simulink model "pompa_cu_perturbatie"  (R2022b)
settings: Solver=VariableStepAuto  StartTime=0.0  StopTime=10.0  RelTol=1e-3
values from neighbouring files (symbols this model uses):
  k = 0.043    [run_first.m]
  k2 = -0.015    [run_first.m]
settings Model: Creator=fabian  LastModifiedBy=fabian

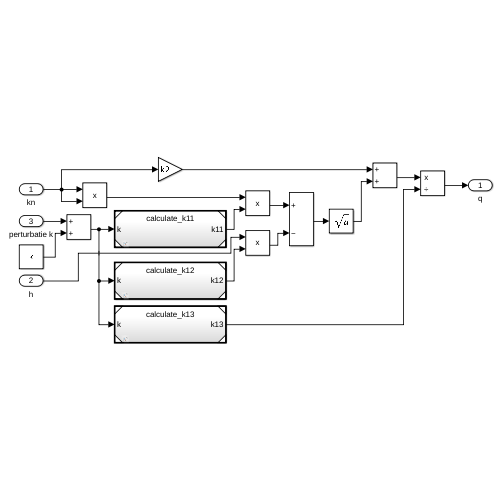
[thumbnail: Simulink's stored preview of the top-level diagram]
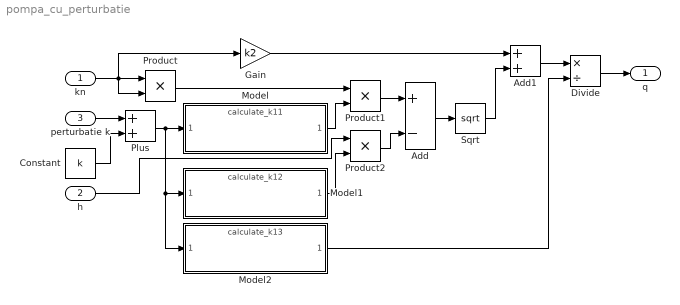
== system pompa_cu_perturbatie ==
  kn : Inport
  h : Inport  Port=2
  perturbatie k : Inport  Port=3
  Add : Sum  Inputs=+-
  Add1 : Sum
  Constant : Constant  Value=k
  Divide : Product  Inputs=*/
  Gain : Gain  Gain=k2
  Model : ModelReference  ModelNameDialog=calculate_k11.slx  SimulationMode=Normal  ModelReferenceVersion=1.1
  Model1 : ModelReference  ModelNameDialog=calculate_k12.slx  SimulationMode=Normal  ModelReferenceVersion=1.1
  Model2 : ModelReference  ModelNameDialog=calculate_k13.slx  SimulationMode=Normal  ModelReferenceVersion=1.1
  Plus : Sum
  Product : Product
  Product1 : Product
  Product2 : Product
  Sqrt : Sqrt
  q : Outport
  wires:
  Gain/1 -> Add1/1
  h/1 -> Product2/1
  Add/1 -> Sqrt/1
  Sqrt/1 -> Add1/2
  Divide/1 -> q/1
  kn/1 -> Gain/1, Product/1, Product/2
  Product1/1 -> Add/1
  Product2/1 -> Add/2
  Product/1 -> Product1/1
  Add1/1 -> Divide/1
  perturbatie k/1 -> Plus/1
  Constant/1 -> Plus/2
  Plus/1 -> Model2/1, Model1/1, Model/1
  Model2/1 -> Divide/2
  Model/1 -> Product1/2
  Model1/1 -> Product2/2
